simulink model "DC_moto_non_linear_model"  (R2025a)
settings: Solver=VariableStepAuto  StartTime=0.0  StopTime=10  RelTol=1e-3
values from neighbouring files (symbols this model uses):
  alfa_ref = 0    [DC_motor_var.mat]    (also in DC_motor_variable.mat)
  D = 0.004    [DC_motor_var.mat]    (also in DC_motor_variable.mat)
  i_initial = 0.04    [DC_motor_var.mat]    (also in DC_motor_variable.mat)
  J = 0.0007046    [DC_motor_var.mat]    (also in DC_motor_variable.mat)
  jurk_ref = 0    [DC_motor_var.mat]    (also in DC_motor_variable.mat)
  Kt = 0.1236    [DC_motor_var.mat]    (also in DC_motor_variable.mat)
  L = 0.917    [DC_motor_var.mat]    (also in DC_motor_variable.mat)
  load_t = 0    [DC_motor_var.mat]    (also in DC_motor_variable.mat)
  q1 = 100    [DC_motor_var.mat]
  q2 = 100    [DC_motor_var.mat]
  q3 = 100    [DC_motor_var.mat]
  R = 7.2    [DC_motor_var.mat]    (also in DC_motor_variable.mat)
  r1 = 10    [DC_motor_var.mat]    (also in DC_motor_variable.mat)
  r2 = 10    [DC_motor_var.mat]    (also in DC_motor_variable.mat)
  r3 = 10    [DC_motor_var.mat]    (also in DC_motor_variable.mat)
  w_ref = 100    [DC_motor_var.mat]    (also in DC_motor_variable.mat = 50)
settings Model: Creator=raja  LastModifiedBy=raja

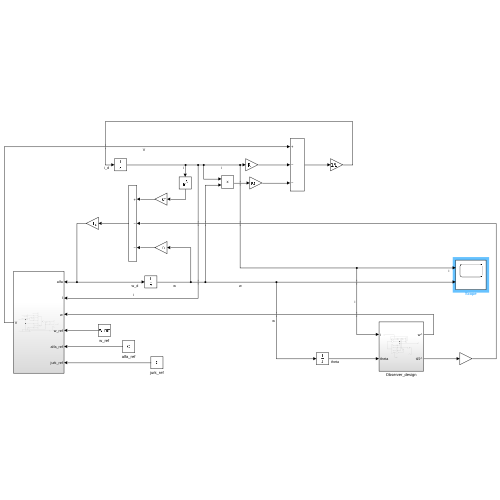
[thumbnail: Simulink's stored preview of the top-level diagram]
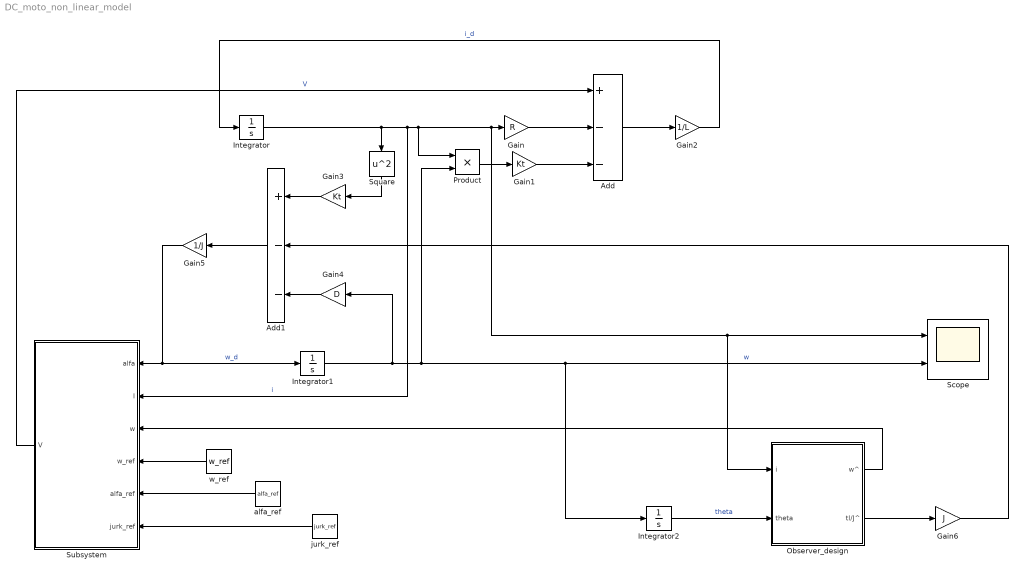
== system DC_moto_non_linear_model ==
  Add : Sum  Inputs=+--
  Add1 : Sum  Inputs=+--
  Gain : Gain  Gain=R
  Gain1 : Gain  Gain=Kt
  Gain2 : Gain  Gain=1/L
  Gain3 : Gain  Gain=Kt
  Gain4 : Gain  Gain=D
  Gain5 : Gain  Gain=1/J
  Gain6 : Gain  Gain=J
  Integrator : Integrator  InitialCondition=i_initial
  Integrator1 : Integrator
  Integrator2 : Integrator
  Observer_design : Subsystem
  Product : Product
  Scope : Scope  NumInputPorts=2
      settings: ActiveDisplayYMinimum=-15.599588809396854  ActiveDisplayYMaximum=140.39629928457171
  Square : Math  Operator=square
  Subsystem : Subsystem
  alfa_ref : Constant  Value=alfa_ref
  jurk_ref : Constant  Value=jurk_ref
  w_ref : Constant  Value=w_ref
  wires:
  Gain2/1 -> Integrator/1  "i_d"
  Integrator/1 -> Subsystem/2(I), Observer_design/1(i), Scope/1, Gain/1, Product/1, Square/1  "i"
  Gain5/1 -> Integrator1/1, Subsystem/1(alfa)  "w_d"
  Integrator1/1 -> Gain4/1, Product/2, Integrator2/1, Scope/2  "w"
  Product/1 -> Gain1/1
  Gain/1 -> Add/2
  Gain1/1 -> Add/3
  Add/1 -> Gain2/1
  Square/1 -> Gain3/1
  Gain3/1 -> Add1/1
  Gain4/1 -> Add1/3
  Gain6/1 -> Add1/2
  Add1/1 -> Gain5/1
  Subsystem/1(V) -> Add/1  "V"
  alfa_ref/1 -> Subsystem/5(alfa_ref)
  w_ref/1 -> Subsystem/4(w_ref)
  jurk_ref/1 -> Subsystem/6(jurk_ref)
  Integrator2/1 -> Observer_design/2(theta)  "theta"
  Observer_design/1(w^) -> Subsystem/3(w)
  Observer_design/2(tl/J^) -> Gain6/1

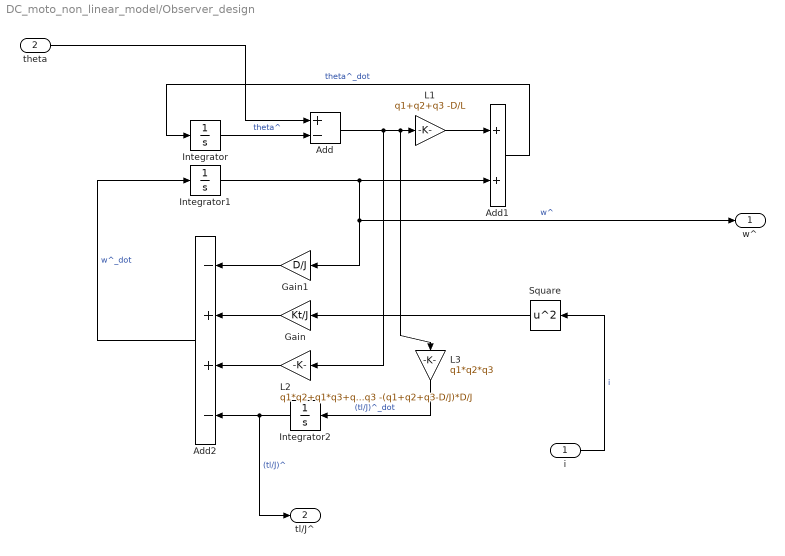
== system DC_moto_non_linear_model/Observer_design ==
  i : Inport
  theta : Inport  Port=2
  Add : Sum  Inputs=+-
  Add1 : Sum
  Add2 : Sum  Inputs=-++-
  Gain : Gain  Gain=Kt/J
  Gain1 : Gain  Gain=D/J
  Integrator : Integrator
  Integrator1 : Integrator
  Integrator2 : Integrator  InitialCondition=load_t/J
  L1 : Gain  Gain=q1+q2+q3 -D/L
  L2 : Gain  Gain=q1*q2+q1*q3+q2*q3 -(q1+q2+q3-D/J)*D/J
  L3 : Gain  Gain=q1*q2*q3
  Square : Math  Operator=square
  w^ : Outport
  tl/J^ : Outport  Port=2
  wires:
  Add1/1 -> Integrator/1  "theta^_dot"
  Integrator/1 -> Add/2  "theta^"
  Add2/1 -> Integrator1/1  "w^_dot"
  Integrator1/1 -> Gain1/1, w^/1, Add1/2  "w^"
  Integrator2/1 -> tl/J^/1, Add2/4  "(tl/J)^"
  theta/1 -> Add/1
  Add/1 -> L2/1, L3/1, L1/1
  L1/1 -> Add1/1
  i/1 -> Square/1  "i"
  Square/1 -> Gain/1
  Gain/1 -> Add2/2
  Gain1/1 -> Add2/1
  L2/1 -> Add2/3
  L3/1 -> Integrator2/1  "(tl/J)^_dot"

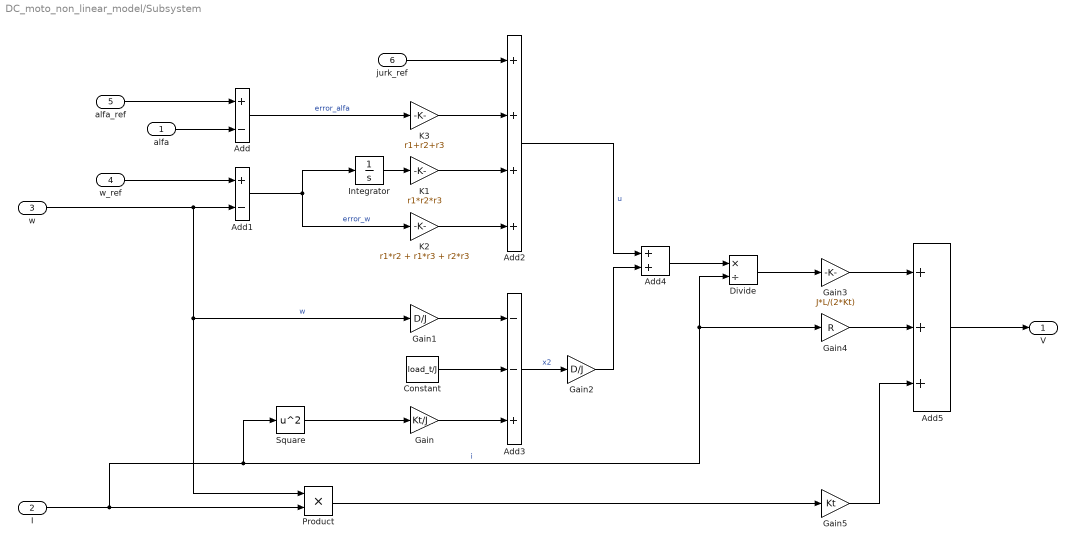
== system DC_moto_non_linear_model/Subsystem ==
  alfa : Inport
  I : Inport  Port=2
  w : Inport  Port=3
  w_ref : Inport  Port=4
  alfa_ref : Inport  Port=5
  jurk_ref : Inport  Port=6
  Add : Sum  Inputs=+-
  Add1 : Sum  Inputs=+-
  Add2 : Sum  Inputs=++++
  Add3 : Sum  Inputs=--+
  Add4 : Sum
  Add5 : Sum  Inputs=+++
  Constant : Constant  Value=load_t/J
  Divide : Product  Inputs=*/
  Gain : Gain  Gain=Kt/J
  Gain1 : Gain  Gain=D/J
  Gain2 : Gain  Gain=D/J
  Gain3 : Gain  Gain=J*L/(2*Kt)
  Gain4 : Gain  Gain=R
  Gain5 : Gain  Gain=Kt
  Integrator : Integrator
  K1 : Gain  Gain=r1*r2*r3
  K2 : Gain  Gain=r1*r2 + r1*r3 + r2*r3
  K3 : Gain  Gain=r1+r2+r3
  Product : Product
  Square : Math  Operator=square
  V : Outport
  wires:
  alfa_ref/1 -> Add/1
  alfa/1 -> Add/2
  w/1 -> Product/1, Gain1/1, Add1/2  "w"
  w_ref/1 -> Add1/1
  Add/1 -> K3/1  "error_alfa"
  Add1/1 -> K2/1, Integrator/1  "error_w"
  Integrator/1 -> K1/1
  jurk_ref/1 -> Add2/1
  K3/1 -> Add2/2
  K1/1 -> Add2/3
  K2/1 -> Add2/4
  Add2/1 -> Add4/1  "u"
  I/1 -> Product/2, Square/1, Divide/2, Gain4/1  "i"
  Square/1 -> Gain/1
  Gain1/1 -> Add3/1
  Constant/1 -> Add3/2
  Gain/1 -> Add3/3
  Add3/1 -> Gain2/1  "x2"
  Gain2/1 -> Add4/2
  Add4/1 -> Divide/1
  Divide/1 -> Gain3/1
  Product/1 -> Gain5/1
  Gain3/1 -> Add5/1
  Gain4/1 -> Add5/2
  Gain5/1 -> Add5/3
  Add5/1 -> V/1
